simulink model "finalcode"  (R2020a)
settings: Solver=FixedStepDiscrete  StartTime=0.0  StopTime=1  FixedStep=0.0005  RelTol=1e-3  EnableMultiTasking=on
undefined symbols (not defined in the file): acc_calmax1, acc_calmax2, acc_calmin1, acc_calmin2, akemancanshu, angle_middle, bre, bre_calmax, bre_calmin, chasuniujvvvv_hou, chasuniujvvvv_qian, chasuuuu, ecucoder_acal, I_AN01_5K1, I_AN03_5V, I_AN04_5V, kd, kddd, ki, kiii, kp, kppp, leftmax, O_SW06_HS1A, P11111, P22222, PIDmodel, PPPP, rightmax, slip, slip_big, slip_little, slipmodel, T_add, T_del, tiaoshi, TTTTTyouren, vvvv, zhiling
libraries: ec5744lib x305, canmsglib x97, simulink x23
(part 4 of 11)

== system finalcode/Subsystem/Rx/惯导/Subsystem2/Subsystem ==
  ID : Inport
  msg : Inport  Port=2
  Enable : EnablePort
  CAN Pack : canmsglib/CAN Pack  Commented=on  CANdbFile=D:\desktop\enable.dbc  MsgList=(none)  MsgName=AMK_ActualValue1  MsgIDType=Standard (11-bit identifier)  MsgIdentifier=643  MsgLength=8  Remote=off  ApplyMinMax=off  BusOutput=off  SignalInfo={'AMK_ActualVelocity','16','16','LE','signed','Standard','0','1','0','0','65535';'AMK_MagnetizingCurrent','48','16','LE','signed','Standard','0','1','0','0','65535';'AMK_TorqueCurrent','32','16','LE','signed','Standard','0','1','0','0','65535';'AMK_bDcOn1','12','1','LE','unsigned','Standard','0','1','0','0','1';'AMK_bDerating1','15','1','LE','unsigned','Standard','0','1','0','0','1';'AMK_bError1','9','1','LE','unsigned','Standard','0','1','0','0','1';'AMK_bInverterOn1','14','1','LE','unsigned','Standard','0','1','0','0','1';'AMK_bQuitDcOn1','11','1','LE','unsigned','Standard','0','1','0','0','1';'AMK_bQuitInverterOn1','13','1','LE','unsigned','Standard','0','1','0','0','1';'AMK_bReserve1','0','8','LE','unsigned','Standard','0','1','0','0','255';'AMK_bSystemReady1','8','1','LE','unsigned','Standard','0','1','0','0','1';'AMK_bWarn1','10','1','LE','unsigned','Standard','0','1','0','0','1'}
      settings: SourceProductBaseCode=ME,XP,VN  DataFormat=CANdb specified signals
  CAN Unpack : canmsglib/CAN Unpack  CANdbFile=C:\Users\Liu keliang\Desktop\HRT2023\HRT23赛季刘科良\CANdbc\homework1.dbc  MsgList=(none)  MsgName=INS_Acc  MsgIDType=Standard (11-bit identifier)  MsgIdentifier=1280  MsgLength=7  SignalInfo={'ACC_X','16','16','BE','unsigned','Standard','0','0.000122','-4','-4','4';'ACC_Y','32','16','BE','unsigned','Standard','0','0.000122','-4','-4','4';'ACC_Z','48','16','BE','unsigned','Standard','0','0.000122','-4','-4','4'}  IDPort=off  TimestampPort=off  ErrorPort=off  RemotePort=off  LengthPort=off  StatusPort=off  ApplyMinMax=off
      settings: SourceProductBaseCode=ME,XP,VN  DataFormat=CANdb specified signals
  CANPackMessage : ec5744lib/RapidECU_U4B/04CANCommunication/CANPackMessage  Commented=on  datalength=8  sampletime=-1
      settings: SourceProductName=ECUCoder for MPC5744
  CANUnPackMessage : ec5744lib/RapidECU_U4B/04CANCommunication/CANUnPackMessage  datalength=7  canmessagetype=Standard(11-bit ID)  sampletime=-1
      settings: SourceProductName=ECUCoder for MPC5744
  wires:
  msg/1 -> CANUnPackMessage/2
  CANUnPackMessage/1 -> CAN Unpack/1
  ID/1 -> CANUnPackMessage/1
  CANPackMessage/1 -> ?
  CAN Pack/1 -> CANPackMessage/1

== system finalcode/Subsystem/Rx/惯导/Subsystem3/Subsystem ==
  ID : Inport
  msg : Inport  Port=2
  Enable : EnablePort
  CAN Pack : canmsglib/CAN Pack  Commented=on  CANdbFile=D:\desktop\enable.dbc  MsgList=(none)  MsgName=AMK_ActualValue1  MsgIDType=Standard (11-bit identifier)  MsgIdentifier=643  MsgLength=8  Remote=off  ApplyMinMax=off  BusOutput=off  SignalInfo={'AMK_ActualVelocity','16','16','LE','signed','Standard','0','1','0','0','65535';'AMK_MagnetizingCurrent','48','16','LE','signed','Standard','0','1','0','0','65535';'AMK_TorqueCurrent','32','16','LE','signed','Standard','0','1','0','0','65535';'AMK_bDcOn1','12','1','LE','unsigned','Standard','0','1','0','0','1';'AMK_bDerating1','15','1','LE','unsigned','Standard','0','1','0','0','1';'AMK_bError1','9','1','LE','unsigned','Standard','0','1','0','0','1';'AMK_bInverterOn1','14','1','LE','unsigned','Standard','0','1','0','0','1';'AMK_bQuitDcOn1','11','1','LE','unsigned','Standard','0','1','0','0','1';'AMK_bQuitInverterOn1','13','1','LE','unsigned','Standard','0','1','0','0','1';'AMK_bReserve1','0','8','LE','unsigned','Standard','0','1','0','0','255';'AMK_bSystemReady1','8','1','LE','unsigned','Standard','0','1','0','0','1';'AMK_bWarn1','10','1','LE','unsigned','Standard','0','1','0','0','1'}
      settings: SourceProductBaseCode=ME,XP,VN  DataFormat=CANdb specified signals
  CAN Unpack : canmsglib/CAN Unpack  CANdbFile=C:\Users\Liu keliang\Desktop\HRT2023\HRT23赛季刘科良\CANdbc\homework1.dbc  MsgList=(none)  MsgName=INS_Speed  MsgIDType=Standard (11-bit identifier)  MsgIdentifier=1285  MsgLength=7  SignalInfo={'INS_EastSpd','32','16','BE','unsigned','Standard','0','0.0030517','-100','-100','100';'INS_NorthSpd','16','16','BE','unsigned','Standard','0','0.0030517','-100','-100','100';'INS_ToGroundSpd','48','16','BE','unsigned','Standard','0','0.0030517','-100','-100','100'}  IDPort=off  TimestampPort=off  ErrorPort=off  RemotePort=off  LengthPort=off  StatusPort=off  ApplyMinMax=off
      settings: SourceProductBaseCode=ME,XP,VN  DataFormat=CANdb specified signals
  CANPackMessage : ec5744lib/RapidECU_U4B/04CANCommunication/CANPackMessage  Commented=on  datalength=8  sampletime=-1
      settings: SourceProductName=ECUCoder for MPC5744
  CANUnPackMessage : ec5744lib/RapidECU_U4B/04CANCommunication/CANUnPackMessage  datalength=7  canmessagetype=Standard(11-bit ID)  sampletime=-1
      settings: SourceProductName=ECUCoder for MPC5744
  wires:
  msg/1 -> CANUnPackMessage/2
  CANUnPackMessage/1 -> CAN Unpack/1
  ID/1 -> CANUnPackMessage/1
  CANPackMessage/1 -> ?
  CAN Pack/1 -> CANPackMessage/1

== system finalcode/Subsystem/Rx/转向——receive编码器/Subsystem3/Subsystem ==
  ID : Inport
  msg : Inport  Port=2
  Enable : EnablePort
  CAN Pack3 : canmsglib/CAN Pack  CANdbFile=C:\Users\86155\Desktop\HRT2024\qkx\can\zhuanjiaobianmaqi.dbc  MsgList=New_Message_1  MsgName=New_Message_1  MsgIDType=Standard (11-bit identifier)  MsgIdentifier=8  MsgLength=8  Remote=off  ApplyMinMax=off  BusOutput=off  SignalInfo={'no_means','0','24','LE','signed','Standard','0','1','0','-Inf','Inf';'steer','24','16','LE','unsigned','Standard','0','0.35156','0','-Inf','Inf'}
      settings: SourceProductBaseCode=ME,XP,VN  DataFormat=CANdb specified signals
  CAN Unpack : canmsglib/CAN Unpack  CANdbFile=C:\Users\86155\Desktop\HRT2024\qkx\can\zhuanjiaobianmaqi.dbc  MsgList=New_Message_1  MsgName=New_Message_1  MsgIDType=Standard (11-bit identifier)  MsgIdentifier=8  MsgLength=8  SignalInfo={'no_means','0','24','LE','signed','Standard','0','1','0','-Inf','Inf';'steer','24','16','LE','unsigned','Standard','0','0.35156','0','-Inf','Inf'}  IDPort=off  TimestampPort=off  ErrorPort=off  RemotePort=off  LengthPort=off  StatusPort=off  ApplyMinMax=off
      settings: SourceProductBaseCode=ME,XP,VN  DataFormat=CANdb specified signals
  CANPackMessage2 : ec5744lib/RapidECU_U4B/04CANCommunication/CANPackMessage  datalength=8  sampletime=-1
      settings: SourceProductName=ECUCoder for MPC5744
  CANTransmit2 : ec5744lib/RapidECU_U4B/04CANCommunication/CANTransmit  canmodule=2  canbuffer=63  canmessageid=hex2dec('08')  canmessagetype=Standard(11-bit ID)  datalength=8  sampletime=-1
      settings: SourceProductName=ECUCoder for MPC5744
  CANUnPackMessage : ec5744lib/RapidECU_U4B/04CANCommunication/CANUnPackMessage  datalength=8  canmessagetype=Standard(11-bit ID)  sampletime=-1
      settings: SourceProductName=ECUCoder for MPC5744
  Data Store Write : DataStoreWrite  DataStoreName=zhuanjiaobianmaqi
  Data Store Write1 : DataStoreWrite  DataStoreName=zhuanjiao_1
  MATLAB Function : MATLAB Function  TreatAsAtomicUnit=on
  MeaModule1 : ec5744lib/RapidECU_U4B/07Calibration/MeaModule  signal=steer_bianmaqi_origin
      settings: SourceProductName=ECUCoder for MPC5744
  MeaModule2 : ec5744lib/RapidECU_U4B/07Calibration/MeaModule  signal=steer_bianmaqi
      settings: SourceProductName=ECUCoder for MPC5744
  Terminator2 : Terminator
  wires:
  msg/1 -> CANUnPackMessage/2
  CANUnPackMessage/1 -> CAN Unpack/1
  ID/1 -> CANUnPackMessage/1
  CAN Unpack/2 -> MeaModule1/1, CAN Pack3/2, MATLAB Function/1(u)
  MATLAB Function/1(y) -> MeaModule2/1
  MeaModule2/1 -> Data Store Write/1
  MeaModule1/1 -> Data Store Write1/1
  CANTransmit2/1 -> Terminator2/1
  CANPackMessage2/1 -> CANTransmit2/1
  CAN Pack3/1 -> CANPackMessage2/1
  CAN Unpack/1 -> CAN Pack3/1

== system finalcode/Subsystem/Rx/转向电机/Subsystem1/Subsystem ==
  ID : Inport
  msg : Inport  Port=2
  Enable : EnablePort
  CAN Pack : canmsglib/CAN Pack  Commented=on  CANdbFile=C:\Users\Liu keliang\Desktop\HRT2023\HRT23赛季刘科良\CANdbc\workstation.dbc  MsgList=(none)  MsgName=workstation  MsgIDType=Standard (11-bit identifier)  MsgIdentifier=32  MsgLength=5  Remote=off  ApplyMinMax=off  BusOutput=off  SignalInfo={'V','8','8','LE','unsigned','Standard','0','1','0','0','255';'V_Copy_1','16','8','LE','unsigned','Standard','0','1','0','0','255';'controlstart','4','1','LE','unsigned','Standard','0','1','0','-Inf','Inf';'status','0','4','LE','unsigned','Standard','0','1','0','0','15';'steering','24','8','LE','signed','Standard','0','1','0','-128','127';'steering_Copy_1','32','8','LE','signed','Standard','0','1','0','-128','127';'vfeedbackk','40','8','LE','unsigned','Standard','0','1','0','-Inf','Inf'}
      settings: SourceProductBaseCode=ME,XP,VN  DataFormat=CANdb specified signals
  CAN Unpack : canmsglib/CAN Unpack  CANdbFile=C:\Users\Liu keliang\Desktop\HRT2023\HRT23赛季刘科良\CANdbc\zhuanxiangbaocuo.dbc  MsgList=(none)  MsgName=New_Message_1  MsgIDType=Standard (11-bit identifier)  MsgIdentifier=129  MsgLength=1  SignalInfo={'New_Signal_1','0','8','LE','signed','Standard','0','1','0','-Inf','Inf'}  IDPort=off  TimestampPort=off  ErrorPort=off  RemotePort=off  LengthPort=off  StatusPort=off  ApplyMinMax=off
      settings: SourceProductBaseCode=ME,XP,VN  DataFormat=CANdb specified signals
  CANPackMessage : ec5744lib/RapidECU_U4B/04CANCommunication/CANPackMessage  Commented=on  datalength=8  sampletime=-1
      settings: SourceProductName=ECUCoder for MPC5744
  CANUnPackMessage : ec5744lib/RapidECU_U4B/04CANCommunication/CANUnPackMessage  datalength=1  canmessagetype=Standard(11-bit ID)  sampletime=-1
      settings: SourceProductName=ECUCoder for MPC5744
  wires:
  msg/1 -> CANUnPackMessage/2
  CANUnPackMessage/1 -> CAN Unpack/1
  ID/1 -> CANUnPackMessage/1
  CANPackMessage/1 -> ?
  CAN Pack/1 -> CANPackMessage/1

== system finalcode/Subsystem/Rx/转向电机/Subsystem3/Subsystem ==
  ID : Inport
  msg : Inport  Port=2
  Enable : EnablePort
  CAN Pack : canmsglib/CAN Pack  Commented=on  CANdbFile=C:\Users\Liu keliang\Desktop\HRT2023\HRT23赛季刘科良\CANdbc\workstation.dbc  MsgList=(none)  MsgName=workstation  MsgIDType=Standard (11-bit identifier)  MsgIdentifier=32  MsgLength=5  Remote=off  ApplyMinMax=off  BusOutput=off  SignalInfo={'V','8','8','LE','unsigned','Standard','0','1','0','0','255';'V_Copy_1','16','8','LE','unsigned','Standard','0','1','0','0','255';'controlstart','4','1','LE','unsigned','Standard','0','1','0','-Inf','Inf';'status','0','4','LE','unsigned','Standard','0','1','0','0','15';'steering','24','8','LE','signed','Standard','0','1','0','-128','127';'steering_Copy_1','32','8','LE','signed','Standard','0','1','0','-128','127';'vfeedbackk','40','8','LE','unsigned','Standard','0','1','0','-Inf','Inf'}
      settings: SourceProductBaseCode=ME,XP,VN  DataFormat=CANdb specified signals
  CAN Unpack : canmsglib/CAN Unpack  CANdbFile=C:\Users\Liu keliang\Desktop\HRT2023\HRT23赛季刘科良\CANdbc\steering.dbc  MsgList=(none)  MsgName=steeringfeedback  MsgIDType=Standard (11-bit identifier)  MsgIdentifier=1153  MsgLength=6  SignalInfo={'konghzizi1','0','8','LE','signed','Standard','0','1','0','-Inf','Inf';'konghzizi1_Copy_1','8','8','LE','signed','Standard','0','1','0','-Inf','Inf';'targetposition','16','32','LE','signed','Standard','0','1','0','0','65535'}  IDPort=off  TimestampPort=off  ErrorPort=off  RemotePort=off  LengthPort=off  StatusPort=off  ApplyMinMax=off
      settings: SourceProductBaseCode=ME,XP,VN  DataFormat=CANdb specified signals
  CANPackMessage : ec5744lib/RapidECU_U4B/04CANCommunication/CANPackMessage  Commented=on  datalength=8  sampletime=-1
      settings: SourceProductName=ECUCoder for MPC5744
  CANUnPackMessage : ec5744lib/RapidECU_U4B/04CANCommunication/CANUnPackMessage  datalength=6  canmessagetype=Standard(11-bit ID)  sampletime=-1
      settings: SourceProductName=ECUCoder for MPC5744
  Data Store Write : DataStoreWrite  DataStoreName=steeringangle
  MATLAB Function : MATLAB Function  TreatAsAtomicUnit=on
  MeaModule8 : ec5744lib/RapidECU_U4B/07Calibration/MeaModule  signal=zhuanxiangdianji
      settings: SourceProductName=ECUCoder for MPC5744
  wires:
  msg/1 -> CANUnPackMessage/2
  CANUnPackMessage/1 -> CAN Unpack/1
  ID/1 -> CANUnPackMessage/1
  CANPackMessage/1 -> ?
  CAN Pack/1 -> CANPackMessage/1
  CAN Unpack/3 -> MeaModule8/1
  MATLAB Function/1(y) -> Data Store Write/1
  MeaModule8/1 -> MATLAB Function/1(u)

== system finalcode/Subsystem/Tx/TX控制器/Subsystem1/算术平均值滤波 ArithmeticAverage ==
  In1 : Inport
  Constant : Constant  Value=10
  Divide : Product  Inputs=*/
  Sum of Elements : Sum  Inputs=+
  Tapped Delay : simulink/Discrete/Tapped Delay  vinit=0.0  samptime=-1  NumDelays=10  DelayOrder=Oldest  includeCurrent=off
  angle : Outport
  wires:
  Tapped Delay/1 -> Sum of Elements/1
  In1/1 -> Tapped Delay/1
  Divide/1 -> angle/1
  Sum of Elements/1 -> Divide/1
  Constant/1 -> Divide/2

== system finalcode/Subsystem/Tx/TX控制器/Subsystem1/算术平均值滤波 ArithmeticAverage1 ==
  In1 : Inport
  Constant : Constant  Value=10
  Divide : Product  Inputs=*/
  Sum of Elements : Sum  Inputs=+
  Tapped Delay : simulink/Discrete/Tapped Delay  vinit=0.0  samptime=-1  NumDelays=10  DelayOrder=Oldest  includeCurrent=off
  angle : Outport
  wires:
  Tapped Delay/1 -> Sum of Elements/1
  In1/1 -> Tapped Delay/1
  Divide/1 -> angle/1
  Sum of Elements/1 -> Divide/1
  Constant/1 -> Divide/2

== system finalcode/Subsystem/Tx/TX控制器/Subsystem1/算术平均值滤波 ArithmeticAverage2 ==
  In1 : Inport
  Constant : Constant  Value=10
  Divide : Product  Inputs=*/
  Sum of Elements : Sum  Inputs=+
  Tapped Delay : simulink/Discrete/Tapped Delay  vinit=0.0  samptime=-1  NumDelays=10  DelayOrder=Oldest  includeCurrent=off
  angle : Outport
  wires:
  Tapped Delay/1 -> Sum of Elements/1
  In1/1 -> Tapped Delay/1
  Divide/1 -> angle/1
  Sum of Elements/1 -> Divide/1
  Constant/1 -> Divide/2

== system finalcode/Subsystem/Tx/TX控制器/Subsystem1/算术平均值滤波 ArithmeticAverage3 ==
  In1 : Inport
  Constant : Constant  Value=10
  Divide : Product  Inputs=*/
  Sum of Elements : Sum  Inputs=+
  Tapped Delay : simulink/Discrete/Tapped Delay  vinit=0.0  samptime=-1  NumDelays=10  DelayOrder=Oldest  includeCurrent=off
  angle : Outport
  wires:
  Tapped Delay/1 -> Sum of Elements/1
  In1/1 -> Tapped Delay/1
  Divide/1 -> angle/1
  Sum of Elements/1 -> Divide/1
  Constant/1 -> Divide/2

== system finalcode/Subsystem/Tx/TX控制器/Subsystem1/算术平均值滤波 ArithmeticAverage4 ==
  In1 : Inport
  Constant : Constant  Value=10
  Divide : Product  Inputs=*/
  Sum of Elements : Sum  Inputs=+
  Tapped Delay : simulink/Discrete/Tapped Delay  vinit=0.0  samptime=-1  NumDelays=10  DelayOrder=Oldest  includeCurrent=off
  angle : Outport
  wires:
  Tapped Delay/1 -> Sum of Elements/1
  In1/1 -> Tapped Delay/1
  Divide/1 -> angle/1
  Sum of Elements/1 -> Divide/1
  Constant/1 -> Divide/2

== system finalcode/Subsystem/Tx/TX控制器/Subsystem1/算术平均值滤波 ArithmeticAverage5 ==
  In1 : Inport
  Constant : Constant  Value=10
  Divide : Product  Inputs=*/
  Sum of Elements : Sum  Inputs=+
  Tapped Delay : simulink/Discrete/Tapped Delay  vinit=0.0  samptime=-1  NumDelays=10  DelayOrder=Oldest  includeCurrent=off
  angle : Outport
  wires:
  Tapped Delay/1 -> Sum of Elements/1
  In1/1 -> Tapped Delay/1
  Divide/1 -> angle/1
  Sum of Elements/1 -> Divide/1
  Constant/1 -> Divide/2

== system finalcode/Subsystem/Tx/TX控制器/Subsystem1/算术平均值滤波 ArithmeticAverage6 ==
  In1 : Inport
  Constant : Constant  Value=10
  Divide : Product  Inputs=*/
  Sum of Elements : Sum  Inputs=+
  Tapped Delay : simulink/Discrete/Tapped Delay  vinit=0.0  samptime=-1  NumDelays=10  DelayOrder=Oldest  includeCurrent=off
  angle : Outport
  wires:
  Tapped Delay/1 -> Sum of Elements/1
  In1/1 -> Tapped Delay/1
  Divide/1 -> angle/1
  Sum of Elements/1 -> Divide/1
  Constant/1 -> Divide/2

== system finalcode/Subsystem/Tx/TX控制器/Subsystem1/算术平均值滤波 ArithmeticAverage7 ==
  In1 : Inport
  Constant : Constant  Value=10
  Divide : Product  Inputs=*/
  Sum of Elements : Sum  Inputs=+
  Tapped Delay : simulink/Discrete/Tapped Delay  vinit=0.0  samptime=-1  NumDelays=10  DelayOrder=Oldest  includeCurrent=off
  angle : Outport
  wires:
  Tapped Delay/1 -> Sum of Elements/1
  In1/1 -> Tapped Delay/1
  Divide/1 -> angle/1
  Sum of Elements/1 -> Divide/1
  Constant/1 -> Divide/2

== system finalcode/Subsystem/Tx/TX控制器/扭矩/184左前 ==
  CAN Pack : canmsglib/CAN Pack  CANdbFile=D:\desktop\CANdbc\enable.dbc  MsgList=(none)  MsgName=first_enable  MsgIDType=Standard (11-bit identifier)  MsgIdentifier=388  MsgLength=8  Remote=off  ApplyMinMax=off  BusOutput=off  SignalInfo={'AMK_Reserve','12','4','LE','signed','Standard','0','1','0','0','15';'AMK_TargetVelocity','16','16','LE','signed','Standard','0','1','0','0','65535';'AMK_TorqueLimitNegativ','48','16','LE','signed','Standard','0','1','0','0','65535';'AMK_TorqueLimitPositiv','32','16','LE','signed','Standard','0','1','0','0','65535';'AMK_bEnable','10','1','LE','unsigned','Standard','0','1','0','0','1';'AMK_bErrorReset','11','1','LE','unsigned','Standard','0','1','0','0','1';'AMK_bInverterOn','8','1','LE','unsigned','Standard','0','1','0','0','1';'AMK_bReserve','0','8','LE','unsigned','Standard','0','1','0','0','255';'CAN_bdcon','9','1','LE','unsigned','Standard','0','1','0','0','1'}
      settings: SourceProductBaseCode=ME,XP,VN  DataFormat=CANdb specified signals
  CAN Pack1 : canmsglib/CAN Pack  CANdbFile=D:\desktop\CANdbc\enable.dbc  MsgList=(none)  MsgName=first_enable  MsgIDType=Standard (11-bit identifier)  MsgIdentifier=388  MsgLength=8  Remote=off  ApplyMinMax=off  BusOutput=off  SignalInfo={'AMK_Reserve','12','4','LE','signed','Standard','0','1','0','0','15';'AMK_TargetVelocity','16','16','LE','signed','Standard','0','1','0','0','65535';'AMK_TorqueLimitNegativ','48','16','LE','signed','Standard','0','1','0','0','65535';'AMK_TorqueLimitPositiv','32','16','LE','signed','Standard','0','1','0','0','65535';'AMK_bEnable','10','1','LE','unsigned','Standard','0','1','0','0','1';'AMK_bErrorReset','11','1','LE','unsigned','Standard','0','1','0','0','1';'AMK_bInverterOn','8','1','LE','unsigned','Standard','0','1','0','0','1';'AMK_bReserve','0','8','LE','unsigned','Standard','0','1','0','0','255';'CAN_bdcon','9','1','LE','unsigned','Standard','0','1','0','0','1'}
      settings: SourceProductBaseCode=ME,XP,VN  DataFormat=CANdb specified signals
  CANPackMessage : ec5744lib/RapidECU_U4B/04CANCommunication/CANPackMessage  datalength=8  sampletime=-1
      settings: SourceProductName=ECUCoder for MPC5744
  CANPackMessage1 : ec5744lib/RapidECU_U4B/04CANCommunication/CANPackMessage  datalength=8  sampletime=-1
      settings: SourceProductName=ECUCoder for MPC5744
  CANTransmit : ec5744lib/RapidECU_U4B/04CANCommunication/CANTransmit  canmodule=0  canbuffer=8  canmessageid=hex2dec('184')  canmessagetype=Standard(11-bit ID)  datalength=8  sampletime=-1
      settings: SourceProductName=ECUCoder for MPC5744
  Constant{,1..3,5,7..10,12,14,16..17} (13 alike) : Constant  Value=0  SampleTime=-1
  Constant{6,11,13,15} (4 alike) : Constant  SampleTime=-1
  Constant4 : Constant  Value=20000  SampleTime=-1
  Data Store Read : DataStoreRead  DataStoreName=lcu_enable_184
  Data Store Read1 : DataStoreRead  DataStoreName=Tzuoqian
  Data Store Read2 : DataStoreRead  DataStoreName=lcu_enable_184_1
  Data Store Read4 : DataStoreRead  DataStoreName=yourenniuju
  Data Type Conversion : DataTypeConversion  OutDataTypeStr=uint8
  Data Type Conversion1 : DataTypeConversion  OutDataTypeStr=uint8
  MeaModule : ec5744lib/RapidECU_U4B/07Calibration/MeaModule  signal=T184
      settings: SourceProductName=ECUCoder for MPC5744
  MeaModule1 : ec5744lib/RapidECU_U4B/07Calibration/MeaModule  signal=Tfirst
      settings: SourceProductName=ECUCoder for MPC5744
  Switch : Switch  Criteria=u2 > Threshold  Threshold=0.9
  Switch1 : Switch  Criteria=u2 > Threshold
  Terminator : Terminator
  wires:
  Constant8/1 -> CAN Pack/8
  Constant5/1 -> CAN Pack/5
  Constant/1 -> CAN Pack/1
  Constant9/1 -> CAN Pack/9
  CAN Pack/1 -> CANPackMessage/1
  Constant7/1 -> CAN Pack/7
  Constant1/1 -> CAN Pack/2
  Constant16/1 -> CAN Pack/4
  Constant2/1 -> CAN Pack/3
  Constant6/1 -> CAN Pack/6
  CANTransmit/1 -> MeaModule/1
  MeaModule/1 -> Terminator/1
  Constant14/1 -> CAN Pack1/8
  Constant3/1 -> CAN Pack1/1
  Constant13/1 -> CAN Pack1/7
  CAN Pack1/1 -> CANPackMessage1/1
  Constant12/1 -> CAN Pack1/6
  CANPackMessage1/1 -> Data Type Conversion1/1
  Constant4/1 -> CAN Pack1/2
  Constant15/1 -> CAN Pack1/9
  Constant11/1 -> CAN Pack1/5
  Data Type Conversion1/1 -> Switch/1
  Constant10/1 -> CAN Pack1/3
  Switch/1 -> CANTransmit/1
  CANPackMessage/1 -> Data Type Conversion/1
  Data Type Conversion/1 -> Switch/3
  MeaModule1/1 -> CAN Pack1/4
  Switch1/1 -> MeaModule1/1
  Data Store Read/1 -> Switch1/2
  Constant17/1 -> Switch1/3
  Data Store Read2/1 -> Switch/2
  Data Store Read4/1 -> Switch1/1

== system finalcode/Subsystem/Tx/TX控制器/扭矩/185右前 ==
  CAN Pack : canmsglib/CAN Pack  CANdbFile=D:\desktop\CANdbc\enable - youqian.dbc  MsgList=(none)  MsgName=first_enable  MsgIDType=Standard (11-bit identifier)  MsgIdentifier=389  MsgLength=8  Remote=off  ApplyMinMax=off  BusOutput=off  SignalInfo={'AMK_Reserve','12','4','LE','signed','Standard','0','1','0','0','15';'AMK_TargetVelocity','16','16','LE','signed','Standard','0','1','0','0','65535';'AMK_TorqueLimitNegativ','48','16','LE','signed','Standard','0','1','0','0','65535';'AMK_TorqueLimitPositiv','32','16','LE','signed','Standard','0','1','0','0','65535';'AMK_bEnable','10','1','LE','unsigned','Standard','0','1','0','0','1';'AMK_bErrorReset','11','1','LE','unsigned','Standard','0','1','0','0','1';'AMK_bInverterOn','8','1','LE','unsigned','Standard','0','1','0','0','1';'AMK_bReserve','0','8','LE','unsigned','Standard','0','1','0','0','255';'CAN_bdcon','9','1','LE','unsigned','Standard','0','1','0','0','1'}
      settings: SourceProductBaseCode=ME,XP,VN  DataFormat=CANdb specified signals
  CAN Pack1 : canmsglib/CAN Pack  CANdbFile=D:\desktop\CANdbc\enable - youqian.dbc  MsgList=(none)  MsgName=first_enable  MsgIDType=Standard (11-bit identifier)  MsgIdentifier=389  MsgLength=8  Remote=off  ApplyMinMax=off  BusOutput=off  SignalInfo={'AMK_Reserve','12','4','LE','signed','Standard','0','1','0','0','15';'AMK_TargetVelocity','16','16','LE','signed','Standard','0','1','0','0','65535';'AMK_TorqueLimitNegativ','48','16','LE','signed','Standard','0','1','0','0','65535';'AMK_TorqueLimitPositiv','32','16','LE','signed','Standard','0','1','0','0','65535';'AMK_bEnable','10','1','LE','unsigned','Standard','0','1','0','0','1';'AMK_bErrorReset','11','1','LE','unsigned','Standard','0','1','0','0','1';'AMK_bInverterOn','8','1','LE','unsigned','Standard','0','1','0','0','1';'AMK_bReserve','0','8','LE','unsigned','Standard','0','1','0','0','255';'CAN_bdcon','9','1','LE','unsigned','Standard','0','1','0','0','1'}
      settings: SourceProductBaseCode=ME,XP,VN  DataFormat=CANdb specified signals
  CANPackMessage : ec5744lib/RapidECU_U4B/04CANCommunication/CANPackMessage  datalength=8  sampletime=-1
      settings: SourceProductName=ECUCoder for MPC5744
  CANPackMessage1 : ec5744lib/RapidECU_U4B/04CANCommunication/CANPackMessage  datalength=8  sampletime=-1
      settings: SourceProductName=ECUCoder for MPC5744
  CANTransmit : ec5744lib/RapidECU_U4B/04CANCommunication/CANTransmit  canmodule=0  canbuffer=11  canmessageid=hex2dec('185')  canmessagetype=Standard(11-bit ID)  datalength=8  sampletime=-1
      settings: SourceProductName=ECUCoder for MPC5744
  Constant{,1..3,5,7..10,12,14,16..17} (13 alike) : Constant  Value=0  SampleTime=-1
  Constant{6,11,13,15} (4 alike) : Constant  SampleTime=-1
  Constant4 : Constant  Value=20000  SampleTime=-1
  Data Store Read1 : DataStoreRead  DataStoreName=Tyouqian
  Data Store Read2 : DataStoreRead  DataStoreName=lcu_enable_185
  Data Store Read3 : DataStoreRead  DataStoreName=lcu_enable_185_1
  Data Store Read5 : DataStoreRead  DataStoreName=yourenniuju
  Data Type Conversion : DataTypeConversion  OutDataTypeStr=uint8
  Data Type Conversion1 : DataTypeConversion  OutDataTypeStr=uint8
  MeaModule : ec5744lib/RapidECU_U4B/07Calibration/MeaModule  signal=T185
      settings: SourceProductName=ECUCoder for MPC5744
  MeaModule1 : ec5744lib/RapidECU_U4B/07Calibration/MeaModule  signal=Tforth
      settings: SourceProductName=ECUCoder for MPC5744
  Switch : Switch  Criteria=u2 > Threshold
  Switch1 : Switch  Criteria=u2 > Threshold
  Terminator : Terminator
  wires:
  Constant8/1 -> CAN Pack/8
  Constant5/1 -> CAN Pack/5
  Constant/1 -> CAN Pack/1
  CANPackMessage/1 -> Data Type Conversion/1
  Constant9/1 -> CAN Pack/9
  CAN Pack/1 -> CANPackMessage/1
  Constant7/1 -> CAN Pack/7
  Constant1/1 -> CAN Pack/2
  Constant16/1 -> CAN Pack/4
  Constant2/1 -> CAN Pack/3
  Constant6/1 -> CAN Pack/6
  CANTransmit/1 -> MeaModule/1
  MeaModule/1 -> Terminator/1
  CANPackMessage1/1 -> Data Type Conversion1/1
  Constant3/1 -> CAN Pack1/1
  Constant11/1 -> CAN Pack1/5
  Constant12/1 -> CAN Pack1/6
  Constant13/1 -> CAN Pack1/7
  CAN Pack1/1 -> CANPackMessage1/1
  Constant10/1 -> CAN Pack1/3
  Constant14/1 -> CAN Pack1/8
  Constant4/1 -> CAN Pack1/2
  Constant15/1 -> CAN Pack1/9
  Data Type Conversion1/1 -> Switch/1
  Data Type Conversion/1 -> Switch/3
  Switch/1 -> CANTransmit/1
  Data Store Read3/1 -> Switch/2
  MeaModule1/1 -> CAN Pack1/4
  Switch1/1 -> MeaModule1/1
  Constant17/1 -> Switch1/3
  Data Store Read2/1 -> Switch1/2
  Data Store Read5/1 -> Switch1/1

== system finalcode/Subsystem/Tx/TX控制器/扭矩/188右后 ==
  CAN Pack : canmsglib/CAN Pack  CANdbFile=D:\desktop\CANdbc\enable - zuohou - 副本.dbc  MsgList=(none)  MsgName=first_enable  MsgIDType=Standard (11-bit identifier)  MsgIdentifier=392  MsgLength=8  Remote=off  ApplyMinMax=off  BusOutput=off  SignalInfo={'AMK_Reserve','12','4','LE','signed','Standard','0','1','0','0','15';'AMK_TargetVelocity','16','16','LE','signed','Standard','0','1','0','0','65535';'AMK_TorqueLimitNegativ','48','16','LE','signed','Standard','0','1','0','0','65535';'AMK_TorqueLimitPositiv','32','16','LE','signed','Standard','0','1','0','0','65535';'AMK_bEnable','10','1','LE','unsigned','Standard','0','1','0','0','1';'AMK_bErrorReset','11','1','LE','unsigned','Standard','0','1','0','0','1';'AMK_bInverterOn','8','1','LE','unsigned','Standard','0','1','0','0','1';'AMK_bReserve','0','8','LE','unsigned','Standard','0','1','0','0','255';'CAN_bdcon','9','1','LE','unsigned','Standard','0','1','0','0','1'}
      settings: SourceProductBaseCode=ME,XP,VN  DataFormat=CANdb specified signals
  CAN Pack1 : canmsglib/CAN Pack  CANdbFile=D:\desktop\CANdbc\enable - zuohou - 副本.dbc  MsgList=(none)  MsgName=first_enable  MsgIDType=Standard (11-bit identifier)  MsgIdentifier=392  MsgLength=8  Remote=off  ApplyMinMax=off  BusOutput=off  SignalInfo={'AMK_Reserve','12','4','LE','signed','Standard','0','1','0','0','15';'AMK_TargetVelocity','16','16','LE','signed','Standard','0','1','0','0','65535';'AMK_TorqueLimitNegativ','48','16','LE','signed','Standard','0','1','0','0','65535';'AMK_TorqueLimitPositiv','32','16','LE','signed','Standard','0','1','0','0','65535';'AMK_bEnable','10','1','LE','unsigned','Standard','0','1','0','0','1';'AMK_bErrorReset','11','1','LE','unsigned','Standard','0','1','0','0','1';'AMK_bInverterOn','8','1','LE','unsigned','Standard','0','1','0','0','1';'AMK_bReserve','0','8','LE','unsigned','Standard','0','1','0','0','255';'CAN_bdcon','9','1','LE','unsigned','Standard','0','1','0','0','1'}
      settings: SourceProductBaseCode=ME,XP,VN  DataFormat=CANdb specified signals
  CANPackMessage : ec5744lib/RapidECU_U4B/04CANCommunication/CANPackMessage  datalength=8  sampletime=-1
      settings: SourceProductName=ECUCoder for MPC5744
  CANPackMessage1 : ec5744lib/RapidECU_U4B/04CANCommunication/CANPackMessage  datalength=8  sampletime=-1
      settings: SourceProductName=ECUCoder for MPC5744
  CANTransmit : ec5744lib/RapidECU_U4B/04CANCommunication/CANTransmit  canmodule=0  canbuffer=9  canmessageid=hex2dec('188')  canmessagetype=Standard(11-bit ID)  datalength=8  sampletime=-1
      settings: SourceProductName=ECUCoder for MPC5744
  Constant{,1..3,5,7..10,12,14,17} (12 alike) : Constant  Value=0  SampleTime=-1
  Constant{6,11,13,15} (4 alike) : Constant  SampleTime=-1
  Constant16 : Constant  Value=0
  Constant4 : Constant  Value=20000  SampleTime=-1
  Data Store Read1 : DataStoreRead  DataStoreName=lcu_enable_188
  Data Store Read2 : DataStoreRead  DataStoreName=Tyouhou
  Data Store Read3 : DataStoreRead  DataStoreName=lcu_enable_188_1
  Data Store Read5 : DataStoreRead  DataStoreName=yourenniuju
  Data Type Conversion : DataTypeConversion  OutDataTypeStr=uint8
  Data Type Conversion1 : DataTypeConversion  OutDataTypeStr=uint8
  MeaModule : ec5744lib/RapidECU_U4B/07Calibration/MeaModule  signal=T188
      settings: SourceProductName=ECUCoder for MPC5744
  MeaModule1 : ec5744lib/RapidECU_U4B/07Calibration/MeaModule  signal=Tsecond
      settings: SourceProductName=ECUCoder for MPC5744
  Switch : Switch  Criteria=u2 > Threshold  Threshold=0.9
  Switch1 : Switch  Criteria=u2 > Threshold
  Terminator : Terminator
  wires:
  Constant8/1 -> CAN Pack/8
  Constant5/1 -> CAN Pack/5
  Constant/1 -> CAN Pack/1
  CANPackMessage/1 -> Data Type Conversion/1
  Constant9/1 -> CAN Pack/9
  CAN Pack/1 -> CANPackMessage/1
  Constant7/1 -> CAN Pack/7
  Constant1/1 -> CAN Pack/2
  Constant16/1 -> CAN Pack/4
  Constant2/1 -> CAN Pack/3
  Constant6/1 -> CAN Pack/6
  CANTransmit/1 -> MeaModule/1
  MeaModule/1 -> Terminator/1
  Data Type Conversion1/1 -> Switch/1
  Constant12/1 -> CAN Pack1/6
  Constant10/1 -> CAN Pack1/3
  Constant4/1 -> CAN Pack1/2
  CANPackMessage1/1 -> Data Type Conversion1/1
  Constant14/1 -> CAN Pack1/8
  Constant3/1 -> CAN Pack1/1
  Constant11/1 -> CAN Pack1/5
  CAN Pack1/1 -> CANPackMessage1/1
  Constant15/1 -> CAN Pack1/9
  Constant13/1 -> CAN Pack1/7
  Data Store Read3/1 -> Switch/2
  Data Type Conversion/1 -> Switch/3
  Switch/1 -> CANTransmit/1
  MeaModule1/1 -> CAN Pack1/4
  Constant17/1 -> Switch1/3
  Data Store Read1/1 -> Switch1/2
  Switch1/1 -> MeaModule1/1
  Data Store Read5/1 -> Switch1/1

== system finalcode/Subsystem/Tx/TX控制器/扭矩/189左后 ==
  CAN Pack : canmsglib/CAN Pack  CANdbFile=D:\desktop\CANdbc\enable - youhou -.dbc  MsgList=(none)  MsgName=first_enable  MsgIDType=Standard (11-bit identifier)  MsgIdentifier=393  MsgLength=8  Remote=off  ApplyMinMax=off  BusOutput=off  SignalInfo={'AMK_Reserve','12','4','LE','signed','Standard','0','1','0','0','15';'AMK_TargetVelocity','16','16','LE','signed','Standard','0','1','0','0','65535';'AMK_TorqueLimitNegativ','48','16','LE','signed','Standard','0','1','0','0','65535';'AMK_TorqueLimitPositiv','32','16','LE','signed','Standard','0','1','0','0','65535';'AMK_bEnable','10','1','LE','unsigned','Standard','0','1','0','0','1';'AMK_bErrorReset','11','1','LE','unsigned','Standard','0','1','0','0','1';'AMK_bInverterOn','8','1','LE','unsigned','Standard','0','1','0','0','1';'AMK_bReserve','0','8','LE','unsigned','Standard','0','1','0','0','255';'CAN_bdcon','9','1','LE','unsigned','Standard','0','1','0','0','1'}
      settings: SourceProductBaseCode=ME,XP,VN  DataFormat=CANdb specified signals
  CAN Pack1 : canmsglib/CAN Pack  CANdbFile=D:\desktop\CANdbc\enable - youhou -.dbc  MsgList=(none)  MsgName=first_enable  MsgIDType=Standard (11-bit identifier)  MsgIdentifier=393  MsgLength=8  Remote=off  ApplyMinMax=off  BusOutput=off  SignalInfo={'AMK_Reserve','12','4','LE','signed','Standard','0','1','0','0','15';'AMK_TargetVelocity','16','16','LE','signed','Standard','0','1','0','0','65535';'AMK_TorqueLimitNegativ','48','16','LE','signed','Standard','0','1','0','0','65535';'AMK_TorqueLimitPositiv','32','16','LE','signed','Standard','0','1','0','0','65535';'AMK_bEnable','10','1','LE','unsigned','Standard','0','1','0','0','1';'AMK_bErrorReset','11','1','LE','unsigned','Standard','0','1','0','0','1';'AMK_bInverterOn','8','1','LE','unsigned','Standard','0','1','0','0','1';'AMK_bReserve','0','8','LE','unsigned','Standard','0','1','0','0','255';'CAN_bdcon','9','1','LE','unsigned','Standard','0','1','0','0','1'}
      settings: SourceProductBaseCode=ME,XP,VN  DataFormat=CANdb specified signals
  CANPackMessage : ec5744lib/RapidECU_U4B/04CANCommunication/CANPackMessage  datalength=8  sampletime=-1
      settings: SourceProductName=ECUCoder for MPC5744
  CANPackMessage1 : ec5744lib/RapidECU_U4B/04CANCommunication/CANPackMessage  datalength=8  sampletime=-1
      settings: SourceProductName=ECUCoder for MPC5744
  CANTransmit : ec5744lib/RapidECU_U4B/04CANCommunication/CANTransmit  canmodule=0  canbuffer=10  canmessageid=hex2dec('189')  canmessagetype=Standard(11-bit ID)  datalength=8  sampletime=-1
      settings: SourceProductName=ECUCoder for MPC5744
  Constant{,1..3,5,7..10,12,14,16..17} (13 alike) : Constant  Value=0  SampleTime=-1
  Constant{6,11,13,15} (4 alike) : Constant  SampleTime=-1
  Constant4 : Constant  Value=20000  SampleTime=-1
  Data Store Read1 : DataStoreRead  DataStoreName=Tzuohou
  Data Store Read2 : DataStoreRead  DataStoreName=lcu_enable_189
  Data Store Read3 : DataStoreRead  DataStoreName=lcu_enable_189_1
  Data Store Read5 : DataStoreRead  DataStoreName=yourenniuju
  Data Type Conversion : DataTypeConversion  OutDataTypeStr=uint8
  Data Type Conversion1 : DataTypeConversion  OutDataTypeStr=uint8
  MeaModule : ec5744lib/RapidECU_U4B/07Calibration/MeaModule  signal=T189
      settings: SourceProductName=ECUCoder for MPC5744
  MeaModule1 : ec5744lib/RapidECU_U4B/07Calibration/MeaModule  signal=Tthird
      settings: SourceProductName=ECUCoder for MPC5744
  Switch : Switch  Criteria=u2 > Threshold
  Switch1 : Switch  Criteria=u2 > Threshold
  Terminator : Terminator
  wires:
  Constant8/1 -> CAN Pack/8
  Constant5/1 -> CAN Pack/5
  Constant/1 -> CAN Pack/1
  CANPackMessage/1 -> Data Type Conversion/1
  Constant9/1 -> CAN Pack/9
  CAN Pack/1 -> CANPackMessage/1
  Constant7/1 -> CAN Pack/7
  Constant1/1 -> CAN Pack/2
  Constant16/1 -> CAN Pack/4
  Constant2/1 -> CAN Pack/3
  Constant6/1 -> CAN Pack/6
  CANTransmit/1 -> MeaModule/1
  MeaModule/1 -> Terminator/1
  Constant12/1 -> CAN Pack1/6
  Constant10/1 -> CAN Pack1/3
  Constant14/1 -> CAN Pack1/8
  Constant4/1 -> CAN Pack1/2
  Constant11/1 -> CAN Pack1/5
  Constant13/1 -> CAN Pack1/7
  CANPackMessage1/1 -> Data Type Conversion1/1
  CAN Pack1/1 -> CANPackMessage1/1
  Constant15/1 -> CAN Pack1/9
  Constant3/1 -> CAN Pack1/1
  Data Type Conversion1/1 -> Switch/1
  Data Type Conversion/1 -> Switch/3
  Switch/1 -> CANTransmit/1
  Data Store Read3/1 -> Switch/2
  MeaModule1/1 -> CAN Pack1/4
  Constant17/1 -> Switch1/3
  Data Store Read2/1 -> Switch1/2
  Switch1/1 -> MeaModule1/1
  Data Store Read5/1 -> Switch1/1

== system finalcode/Subsystem/Tx/TX控制器/扭矩/TEST ==
  Data Store Read : DataStoreRead  Commented=on  DataStoreName=match_model
  MATLAB Function : MATLAB Function  Commented=on  TreatAsAtomicUnit=on
  Subsystem : Subsystem  Commented=on
  wires:
  Data Store Read/1 -> MATLAB Function/1(u)
  MATLAB Function/1(y) -> Subsystem/Enable

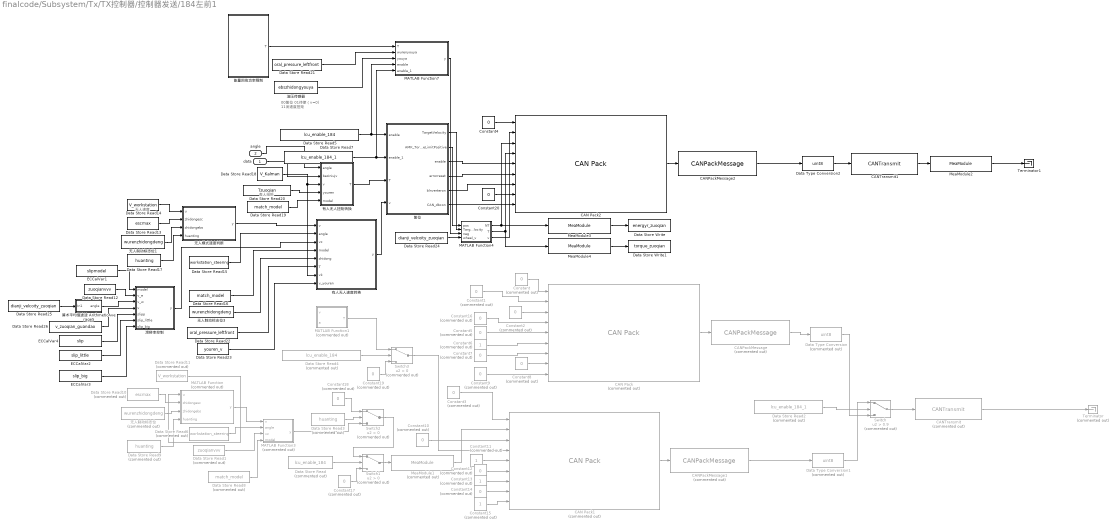
== system finalcode/Subsystem/Tx/TX控制器/控制器发送/184左前1 ==
  note: 无人速度
  note: 有人扭矩
  note: 00复位
      | 01待使（v=0)
      | 11发速度扭矩
  data : Inport
  angle : Inport  Port=2
  CAN Pack : canmsglib/CAN Pack  Commented=on  CANdbFile=D:\desktop\CANdbc\enable.dbc  MsgList=(none)  MsgName=first_enable  MsgIDType=Standard (11-bit identifier)  MsgIdentifier=388  MsgLength=8  Remote=off  ApplyMinMax=off  BusOutput=off  SignalInfo={'AMK_Reserve','12','4','LE','signed','Standard','0','1','0','0','15';'AMK_TargetVelocity','16','16','LE','signed','Standard','0','1','0','0','65535';'AMK_TorqueLimitNegativ','48','16','LE','signed','Standard','0','1','0','0','65535';'AMK_TorqueLimitPositiv','32','16','LE','signed','Standard','0','1','0','0','65535';'AMK_bEnable','10','1','LE','unsigned','Standard','0','1','0','0','1';'AMK_bErrorReset','11','1','LE','unsigned','Standard','0','1','0','0','1';'AMK_bInverterOn','8','1','LE','unsigned','Standard','0','1','0','0','1';'AMK_bReserve','0','8','LE','unsigned','Standard','0','1','0','0','255';'CAN_bdcon','9','1','LE','unsigned','Standard','0','1','0','0','1'}
      settings: SourceProductBaseCode=ME,XP,VN  DataFormat=CANdb specified signals
  CAN Pack1 : canmsglib/CAN Pack  Commented=on  CANdbFile=D:\desktop\CANdbc\enable.dbc  MsgList=(none)  MsgName=first_enable  MsgIDType=Standard (11-bit identifier)  MsgIdentifier=388  MsgLength=8  Remote=off  ApplyMinMax=off  BusOutput=off  SignalInfo={'AMK_Reserve','12','4','LE','signed','Standard','0','1','0','0','15';'AMK_TargetVelocity','16','16','LE','signed','Standard','0','1','0','0','65535';'AMK_TorqueLimitNegativ','48','16','LE','signed','Standard','0','1','0','0','65535';'AMK_TorqueLimitPositiv','32','16','LE','signed','Standard','0','1','0','0','65535';'AMK_bEnable','10','1','LE','unsigned','Standard','0','1','0','0','1';'AMK_bErrorReset','11','1','LE','unsigned','Standard','0','1','0','0','1';'AMK_bInverterOn','8','1','LE','unsigned','Standard','0','1','0','0','1';'AMK_bReserve','0','8','LE','unsigned','Standard','0','1','0','0','255';'CAN_bdcon','9','1','LE','unsigned','Standard','0','1','0','0','1'}
      settings: SourceProductBaseCode=ME,XP,VN  DataFormat=CANdb specified signals
  CAN Pack2 : canmsglib/CAN Pack  CANdbFile=C:\Users\86155\Desktop\HRT2024\qkx\can\enable.dbc  MsgList=(none)  MsgName=first_enable  MsgIDType=Standard (11-bit identifier)  MsgIdentifier=388  MsgLength=8  Remote=off  ApplyMinMax=off  BusOutput=off  SignalInfo={'AMK_Reserve','12','4','LE','signed','Standard','0','1','0','-8','7';'AMK_TargetVelocity','16','16','LE','signed','Standard','0','1','0','-32768','32767';'AMK_TorqueLimitNegativ','48','16','LE','signed','Standard','0','1','0','-32768','32767';'AMK_TorqueLimitPositiv','32','16','LE','signed','Standard','0','1','0','-32768','32767';'AMK_bEnable','10','1','LE','unsigned','Standard','0','1','0','0','1';'AMK_bErrorReset','11','1','LE','unsigned','Standard','0','1','0','0','1';'AMK_bInverterOn','8','1','LE','unsigned','Standard','0','1','0','0','1';'AMK_bReserve','0','8','LE','unsigned','Standard','0','1','0','0','255';'CAN_bdcon','9','1','LE','unsigned','Standard','0','1','0','0','1'}
      settings: SourceProductBaseCode=ME,XP,VN  DataFormat=CANdb specified signals
  CANPackMessage : ec5744lib/RapidECU_U4B/04CANCommunication/CANPackMessage  Commented=on  datalength=8  sampletime=-1
      settings: SourceProductName=ECUCoder for MPC5744
  CANPackMessage1 : ec5744lib/RapidECU_U4B/04CANCommunication/CANPackMessage  Commented=on  datalength=8  sampletime=-1
      settings: SourceProductName=ECUCoder for MPC5744
  CANPackMessage2 : ec5744lib/RapidECU_U4B/04CANCommunication/CANPackMessage  datalength=8  sampletime=-1
      settings: SourceProductName=ECUCoder for MPC5744
  CANTransmit : ec5744lib/RapidECU_U4B/04CANCommunication/CANTransmit  Commented=on  canmodule=0  canbuffer=8  canmessageid=hex2dec('184')  canmessagetype=Standard(11-bit ID)  datalength=8  sampletime=-1
      settings: SourceProductName=ECUCoder for MPC5744
  CANTransmit1 : ec5744lib/RapidECU_U4B/04CANCommunication/CANTransmit  canmodule=0  canbuffer=8  canmessageid=hex2dec('184')  canmessagetype=Standard(11-bit ID)  datalength=8  sampletime=-1
      settings: SourceProductName=ECUCoder for MPC5744
  Constant{,1..3,5,7..10,12,14,16..17,19} (14 alike) : Constant  Commented=on  Value=0  SampleTime=-1
  Constant{6,11,13,15} (4 alike) : Constant  Commented=on  SampleTime=-1
  Constant18 : Constant  Commented=on  Value=0
  Constant20 : Constant  Value=0  SampleTime=-1
  Constant4 : Constant  Value=0  SampleTime=-1
  Data Store Read : DataStoreRead  Commented=on  DataStoreName=lcu_enable_184
  Data Store Read1 : DataStoreRead  Commented=on  DataStoreName=zuoqianvvv
  Data Store Read10 : DataStoreRead  Commented=on  DataStoreName=escmax
  Data Store Read11 : DataStoreRead  Commented=on  DataStoreName=V_workstation
  Data Store Read12 : DataStoreRead  DataStoreName=zuoqianvvv
  Data Store Read13 : DataStoreRead  DataStoreName=escmax
  Data Store Read14 : DataStoreRead  DataStoreName=V_workstation
  Data Store Read15 : DataStoreRead  DataStoreName=workstation_steering
  Data Store Read16 : DataStoreRead  DataStoreName=match_model
  Data Store Read17 : DataStoreRead  DataStoreName=huanting
  Data Store Read18 : DataStoreRead  DataStoreName=V_Kalman
  Data Store Read19 : DataStoreRead  DataStoreName=match_model
  Data Store Read2 : DataStoreRead  Commented=on  DataStoreName=lcu_enable_184_1
  Data Store Read20 : DataStoreRead  DataStoreName=Tzuoqian
  Data Store Read21 : DataStoreRead  DataStoreName=oral_pressure_leftfront
  Data Store Read22 : DataStoreRead  DataStoreName=oral_pressure_leftfront
  Data Store Read23 : DataStoreRead  DataStoreName=youren_v
  Data Store Read24 : DataStoreRead  DataStoreName=dianji_velcoity_zuoqian
  Data Store Read25 : DataStoreRead  DataStoreName=dianji_velcoity_zuoqian
  Data Store Read26 : DataStoreRead  DataStoreName=v_zuoqian_guandao
  Data Store Read3 : DataStoreRead  Commented=on  DataStoreName=huanting
  Data Store Read4 : DataStoreRead  Commented=on  DataStoreName=lcu_enable_184
  Data Store Read5 : DataStoreRead  DataStoreName=lcu_enable_184
  Data Store Read6 : DataStoreRead  Commented=on  DataStoreName=workstation_steering
  Data Store Read7 : DataStoreRead  DataStoreName=lcu_enable_184_1
  Data Store Read8 : DataStoreRead  Commented=on  DataStoreName=match_model
  Data Store Read9 : DataStoreRead  Commented=on  DataStoreName=huanting
  Data Store Write : DataStoreWrite  DataStoreName=energyr_zuoqian
  Data Store Write1 : DataStoreWrite  DataStoreName=torque_zuoqian
  Data Type Conversion : DataTypeConversion  Commented=on  OutDataTypeStr=uint8
  Data Type Conversion1 : DataTypeConversion  Commented=on  OutDataTypeStr=uint8
  Data Type Conversion2 : DataTypeConversion  OutDataTypeStr=uint8
  ECCalVar1 : Constant  InitFcn=ecucoder_acal;  Value=slipmodel  OutDataTypeStr=Inherit: Inherit via back propagation  SampleTime=-1
  ECCalVar2 : Constant  InitFcn=ecucoder_acal;  Value=slip_little  OutDataTypeStr=Inherit: Inherit via back propagation  SampleTime=-1
  ECCalVar3 : Constant  InitFcn=ecucoder_acal;  Value=slip_big  OutDataTypeStr=Inherit: Inherit via back propagation  SampleTime=-1
  ECCalVar4 : Constant  InitFcn=ecucoder_acal;  Value=slip  OutDataTypeStr=Inherit: Inherit via back propagation  SampleTime=-1
  MATLAB Function : MATLAB Function  Commented=on  TreatAsAtomicUnit=on
  MATLAB Function1 : MATLAB Function  Commented=on  TreatAsAtomicUnit=on
  MATLAB Function3 : MATLAB Function  Commented=on  TreatAsAtomicUnit=on
  MATLAB Function4 : MATLAB Function  TreatAsAtomicUnit=on
  MATLAB Function7 : MATLAB Function  TreatAsAtomicUnit=on
  MeaModule1 : ec5744lib/RapidECU_U4B/07Calibration/MeaModule  Commented=on  signal=Vfirst
      settings: SourceProductName=ECUCoder for MPC5744
  MeaModule2 : ec5744lib/RapidECU_U4B/07Calibration/MeaModule  signal=V184
      settings: SourceProductName=ECUCoder for MPC5744
  MeaModule3 : ec5744lib/RapidECU_U4B/07Calibration/MeaModule  signal=NT_zuoqian
      settings: SourceProductName=ECUCoder for MPC5744
  MeaModule4 : ec5744lib/RapidECU_U4B/07Calibration/MeaModule  signal=T_zuoqian
      settings: SourceProductName=ECUCoder for MPC5744
  Switch : Switch  Commented=on  Criteria=u2 > Threshold  Threshold=0.9
  Switch1 : Switch  Commented=on  Criteria=u2 > Threshold
  Switch2 : Switch  Commented=on  Criteria=u2 > Threshold
  Switch3 : Switch  Commented=on  Criteria=u2 > Threshold
  Terminator : Terminator  Commented=on
  Terminator1 : Terminator
  复位 : MATLAB Function  TreatAsAtomicUnit=on
  无人制动标志位 : DataStoreRead  Commented=on  DataStoreName=wurenzhidongdeng
  无人制动标志位1 : DataStoreRead  DataStoreName=wurenzhidongdeng
  无人制动标志位3 : DataStoreRead  DataStoreName=wurenzhidongdeng
  无人模式速度判断 : MATLAB Function  TreatAsAtomicUnit=on
  有人无人扭矩转换 : MATLAB Function  TreatAsAtomicUnit=on
  有人无人速度转换 : MATLAB Function  TreatAsAtomicUnit=on
  油压传感器 : DataStoreRead  DataStoreName=ebszhidongyouya
  滑移率控制 : MATLAB Function  TreatAsAtomicUnit=on
  算术平均值滤波 ArithmeticAverage5 : Subsystem
  能量回收功率限制 : Subsystem
  wires:
  有人无人扭矩转换/1(T) -> 复位/3(T)
  有人无人速度转换/1(y) -> 复位/4(v)
  Data Store Read13/1 -> 无人模式速度判断/2(zhidongesc)
  Data Store Read16/1 -> 有人无人速度转换/4(model)
  Data Store Read15/1 -> 有人无人速度转换/2(angle)
  Data Store Read14/1 -> 无人模式速度判断/1(u)
  无人制动标志位1/1 -> 无人模式速度判断/3(zhidongebs)
  无人模式速度判断/1(y) -> 有人无人速度转换/1(v)
  Data Store Read17/1 -> 无人模式速度判断/4(huanting)
  Data Store Read9/1 -> MATLAB Function/4(huanting)
  Data Store Read7/1 -> MATLAB Function7/5(enable_1), 复位/2(enable_1)
  Data Store Read5/1 -> MATLAB Function7/4(enable), 复位/1("enable ")
  复位/2(AMK_TorqueLimitPositive) -> MATLAB Function4/1(pos)
  复位/6(CAN_dbcon) -> CAN Pack2/9
  复位/5(blnverteron) -> CAN Pack2/7
  复位/4(errorreset) -> CAN Pack2/6
  复位/3(enable) -> CAN Pack2/5
  Constant20/1 -> CAN Pack2/8
  Constant4/1 -> CAN Pack2/1
  Data Type Conversion2/1 -> CANTransmit1/1
  CANTransmit1/1 -> MeaModule2/1
  CANPackMessage2/1 -> Data Type Conversion2/1
  CAN Pack2/1 -> CANPackMessage2/1
  MeaModule2/1 -> Terminator1/1
  Data Store Read1/1 -> MATLAB Function3/3(vz)
  Data Store Read11/1 -> MATLAB Function/1(u)
  无人制动标志位/1 -> MATLAB Function/3(zhidongebs)
  Data Store Read10/1 -> MATLAB Function/2(zhidongesc)
  Data Store Read8/1 -> MATLAB Function3/4(model)
  Data Store Read6/1 -> MATLAB Function3/2(angle)
  MATLAB Function3/1(y) -> Switch2/3
  MATLAB Function/1(y) -> MATLAB Function3/1(v)
  MATLAB Function1/1(T) -> Switch3/1
  Switch3/1 -> CAN Pack1/4
  Constant19/1 -> Switch3/3
  Data Store Read4/1 -> Switch3/2
  MeaModule1/1 -> CAN Pack1/2
  Switch2/1 -> Switch1/1
  Constant18/1 -> Switch2/1
  Data Store Read3/1 -> Switch2/2
  Data Store Read2/1 -> Switch/2
  Constant17/1 -> Switch1/3
  Data Store Read/1 -> Switch1/2
  Switch1/1 -> MeaModule1/1
  Data Type Conversion/1 -> Switch/3
  CANPackMessage/1 -> Data Type Conversion/1
  Switch/1 -> CANTransmit/1
  Constant10/1 -> CAN Pack1/3
  Data Type Conversion1/1 -> Switch/1
  Constant11/1 -> CAN Pack1/5
  Constant15/1 -> CAN Pack1/9
  CANPackMessage1/1 -> Data Type Conversion1/1
  Constant12/1 -> CAN Pack1/6
  CAN Pack1/1 -> CANPackMessage1/1
  Constant13/1 -> CAN Pack1/7
  Constant3/1 -> CAN Pack1/1
  Constant14/1 -> CAN Pack1/8
  CANTransmit/1 -> Terminator/1
  Constant6/1 -> CAN Pack/6
  Constant2/1 -> CAN Pack/3
  Constant16/1 -> CAN Pack/4
  Constant1/1 -> CAN Pack/2
  Constant7/1 -> CAN Pack/7
  CAN Pack/1 -> CANPackMessage/1
  Constant9/1 -> CAN Pack/9
  Constant/1 -> CAN Pack/1
  Constant5/1 -> CAN Pack/5
  Constant8/1 -> CAN Pack/8
  Data Store Read18/1 -> 有人无人速度转换/7(vk), 有人无人扭矩转换/3(v)
  Data Store Read19/1 -> 有人无人扭矩转换/5(model)
  Data Store Read20/1 -> 有人无人扭矩转换/4(youren)
  油压传感器/1 -> MATLAB Function7/3(youya)
  Data Store Read21/1 -> MATLAB Function7/2(wurenyouya)
  无人制动标志位3/1 -> 有人无人速度转换/5(zhidong)
  能量回收功率限制/1(T) -> MATLAB Function7/1(T)
  Data Store Read22/1 -> 有人无人速度转换/6(T)
  MATLAB Function7/1(y) -> MATLAB Function4/3(neg)
  Data Store Read23/1 -> 有人无人速度转换/8(v_youren)
  MATLAB Function4/2(T) -> MeaModule4/1, CAN Pack2/4
  MATLAB Function4/3(v) -> CAN Pack2/2
  复位/1(TargetVelocity) -> MATLAB Function4/2(TargetVelocity)
  Data Store Read24/1 -> MATLAB Function4/4(wheel_v)
  MeaModule4/1 -> Data Store Write1/1
  MeaModule3/1 -> Data Store Write/1
  MATLAB Function4/1(NT) -> MeaModule3/1, CAN Pack2/3
  Data Store Read12/1 -> 滑移率控制/2(v_e)
  Data Store Read25/1 -> 算术平均值滤波 ArithmeticAverage5/1(In1)
  Data Store Read26/1 -> 滑移率控制/4(v)
  算术平均值滤波 ArithmeticAverage5/1(angle) -> 滑移率控制/3(v_w)
  滑移率控制/1(y) -> 有人无人速度转换/3(vz)
  data/1 -> 有人无人扭矩转换/2(baziniujv)
  angle/1 -> 有人无人扭矩转换/1(angle)
  ECCalVar1/1 -> 滑移率控制/1(model)
  ECCalVar2/1 -> 滑移率控制/6(slip_little)
  ECCalVar3/1 -> 滑移率控制/7(slip_big)
  ECCalVar4/1 -> 滑移率控制/5(slipp)
